simulink model "b_SCARA_4_DOF_disturbance"  (R2024b)
settings: Solver=ode45  StartTime=0.0  StopTime=8  RelTol=1e-3
libraries: sm_lib x13, nesl_utility x13
settings Model: Creator=Hamid Reza  LastModifiedBy=Hamid Reza
settings SolverCC: MaxConsecutiveZCs=50000

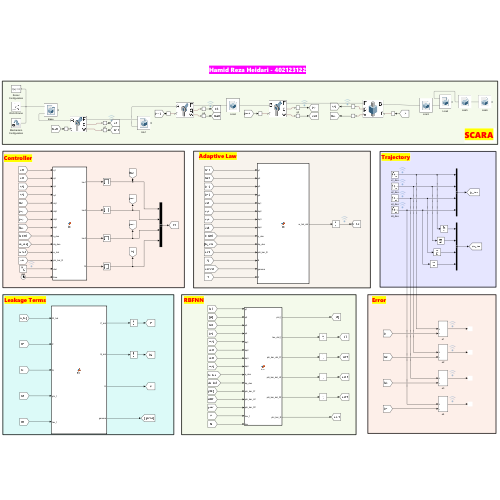
[thumbnail: Simulink's stored preview of the top-level diagram]
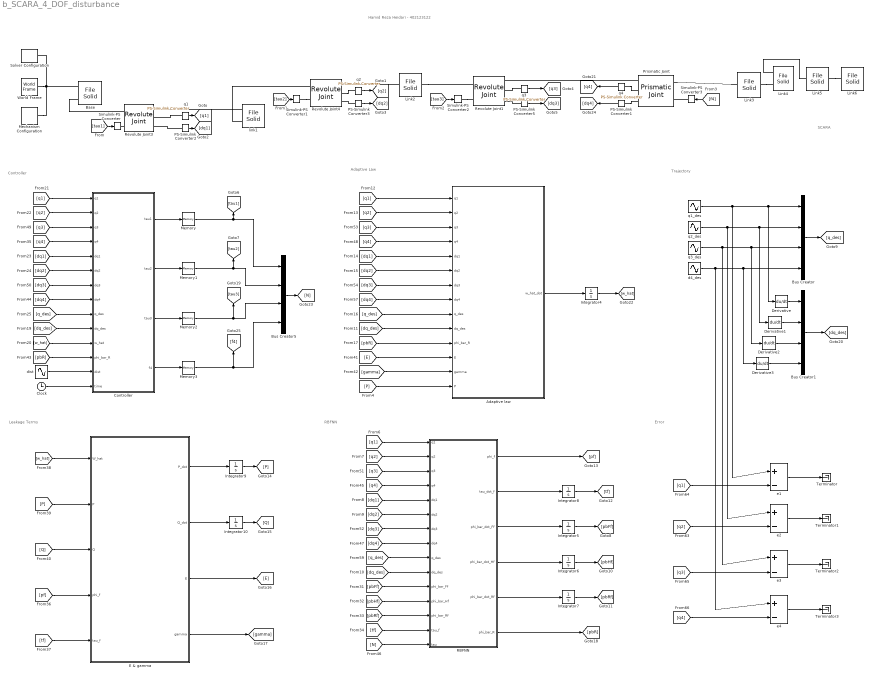
== system b_SCARA_4_DOF_disturbance ==
  note: SCARA
  note: RBFNN
  note: Controller
  note: Adaptive Law
  note: Leakage Terms
  note: Trajectory
  note: Error
  note: Hamid Reza Heidari - 402123122
  Adaptive law : MATLAB Function  TreatAsAtomicUnit=on
  Base : sm_lib/Body Elements/File Solid  ExtGeomFileName=D:\Education\ME\This Semester\Advance Robotics\HW\SimScape\Project 1\SCARA Model_SDLPRT Format\grnd.SLDPRT  UnitType=FromFile  ExtGeomFileUnits=m  StepReaderType=HEX  ExportConvexHullGeometry=off  InertiaType=CalculateFromGeometry  BasedOnType=Mass  Density=1000  DensityUnits=kg/m^3  Mass=5257.95  MassUnits=g  CenterOfMass=[0 0 0]  CenterOfMassUnits=m  MomentsOfInertia=[1 1 1]  MomentsOfInertiaUnits=kg*m^2  ProductsOfInertia=[0 0 0]  ProductsOfInertiaUnits=kg*m^2  GraphicType=FromGeometry  MarkerShape=Sphere  MarkerSize=10  GraphicVisPropType=SimpleVisualProperties  GraphicDiffuseColor=[0.5 0.5 0.5]  GraphicOpacity=1.0  GraphicSpecularColor=[0.5 0.5 0.5 1.0]  GraphicAmbientColor=[0.15 0.15 0.15 1.0]  GraphicEmissiveColor=[0.0 0.0 0.0 1.0]  GraphicShininess=75  DoExposeReferenceFrame=on  SerializedFrames=<Frames><Frame><Id>Frame1</Id><Value><Name>{0}</Name><Origin><Source>GeometricFeature</Source><FeatureName>general surface 32</FeatureName></Origin><PrimaryAxis><DefinedDirection>+X</DefinedDirection><Source>ReferenceFrame</Source><SourceDirection>-Y</SourceDirection><FeatureName></FeatureName></PrimaryAxis><SecondaryAxis><DefinedDirection>+Z</DefinedDirection><Source>ReferenceFrame</Source><SourceDirection>+Z</SourceDirection><FeatureName></FeatureName></SecondaryAxis></Value></Frame><Frame><Id>Frame2</Id><Value><Name>{1}</Name><Origin><Source>GeometricFeature</Source><FeatureName>general surface 10</FeatureName></Origin><PrimaryAxis><DefinedDirection>+Z</DefinedDirection><Source>ReferenceFrame</Source><SourceDirection>+Z</SourceDirection><FeatureName></FeatureName></PrimaryAxis><SecondaryAxis><DefinedDirection>+X</DefinedDirection><Source>ReferenceFrame</Source><SourceDirection>+X</SourceDirection><FeatureName></FeatureName></SecondaryAxis></Value></Frame></Frames>
  Bus Creator : BusCreator  Inputs=4
  Bus Creator1 : BusCreator  Inputs=4
  Bus Creator5 : BusCreator  Inputs=4
  Clock : Clock
  Controller : MATLAB Function  TreatAsAtomicUnit=on
  Derivative{,1..3} (4 alike) : Derivative
  E & gamma : MATLAB Function  TreatAsAtomicUnit=on
  Integrator10 : Integrator  InitialCondition=zeros([4 450])
  Integrator4 : Integrator  InitialCondition=zeros([4 450])  ContinuousStateAttributes='w_hat'
  Integrator5 : Integrator  InitialCondition=zeros([450 1])
  Integrator6 : Integrator  InitialCondition=zeros([450 1])
  Integrator7 : Integrator  InitialCondition=zeros([450 1])
  Integrator8 : Integrator  InitialCondition=zeros([4 1])
  Integrator9 : Integrator  InitialCondition=zeros([450 450])
  Link2 : sm_lib/Body Elements/File Solid  ExtGeomFileName=D:\Education\ME\This Semester\Advance Robotics\HW\SimScape\Project 1\SCARA Model_SDLPRT Format\link2.SLDPRT  UnitType=FromFile  ExtGeomFileUnits=m  StepReaderType=HEX  ExportConvexHullGeometry=off  InertiaType=CalculateFromGeometry  BasedOnType=Mass  Density=1000  DensityUnits=kg/m^3  Mass=5177.21  MassUnits=g  CenterOfMass=[0 0 0]  CenterOfMassUnits=m  MomentsOfInertia=[1 1 1]  MomentsOfInertiaUnits=kg*m^2  ProductsOfInertia=[0 0 0]  ProductsOfInertiaUnits=kg*m^2  GraphicType=FromGeometry  MarkerShape=Sphere  MarkerSize=10  GraphicVisPropType=SimpleVisualProperties  GraphicDiffuseColor=[0.5 0.5 0.5]  GraphicOpacity=1.0  GraphicSpecularColor=[0.5 0.5 0.5 1.0]  GraphicAmbientColor=[0.15 0.15 0.15 1.0]  GraphicEmissiveColor=[0.0 0.0 0.0 1.0]  GraphicShininess=75  DoExposeReferenceFrame=on  SerializedFrames=<Frames><Frame><Id>Frame2</Id><Value><Name>{4}</Name><Origin><Source>GeometricFeature</Source><FeatureName>circular curve 66</FeatureName></Origin><PrimaryAxis><DefinedDirection>+Z</DefinedDirection><Source>ReferenceFrame</Source><SourceDirection>+Z</SourceDirection><FeatureName></FeatureName></PrimaryAxis><SecondaryAxis><DefinedDirection>+X</DefinedDirection><Source>ReferenceFrame</Source><SourceDirection>+X</SourceDirection><FeatureName></FeatureName></SecondaryAxis></Value></Frame></Frames>
  Link3 : sm_lib/Body Elements/File Solid  ExtGeomFileName=D:\Education\ME\This Semester\Advance Robotics\HW\SimScape\Project 1\SCARA Model_SDLPRT Format\link3.SLDPRT  UnitType=FromFile  ExtGeomFileUnits=m  StepReaderType=HEX  ExportConvexHullGeometry=off  InertiaType=CalculateFromGeometry  BasedOnType=Mass  Density=1000  DensityUnits=kg/m^3  Mass=7274.75  MassUnits=g  CenterOfMass=[0 0 0]  CenterOfMassUnits=m  MomentsOfInertia=[1 1 1]  MomentsOfInertiaUnits=kg*m^2  ProductsOfInertia=[0 0 0]  ProductsOfInertiaUnits=kg*m^2  GraphicType=FromGeometry  MarkerShape=Sphere  MarkerSize=10  GraphicVisPropType=SimpleVisualProperties  GraphicDiffuseColor=[0.5 0.5 0.5]  GraphicOpacity=1.0  GraphicSpecularColor=[0.5 0.5 0.5 1.0]  GraphicAmbientColor=[0.15 0.15 0.15 1.0]  GraphicEmissiveColor=[0.0 0.0 0.0 1.0]  GraphicShininess=75  DoExposeReferenceFrame=on  SerializedFrames=<Frames><Frame><Id>Frame2</Id><Value><Name>{5}</Name><Origin><Source>GeometricFeature</Source><FeatureName>general surface 4</FeatureName></Origin><PrimaryAxis><DefinedDirection>+Z</DefinedDirection><Source>ReferenceFrame</Source><SourceDirection>-Z</SourceDirection><FeatureName></FeatureName></PrimaryAxis><SecondaryAxis><DefinedDirection>+X</DefinedDirection><Source>ReferenceFrame</Source><SourceDirection>+X</SourceDirection><FeatureName></FeatureName></SecondaryAxis></Value></Frame></Frames>
  Link4 : sm_lib/Body Elements/File Solid  ExtGeomFileName=D:\Education\ME\This Semester\Advance Robotics\HW\SimScape\Project 1\SCARA Model_SDLPRT Format\link4.SLDPRT  UnitType=FromFile  ExtGeomFileUnits=m  StepReaderType=HEX  ExportConvexHullGeometry=off  InertiaType=CalculateFromGeometry  BasedOnType=Mass  Density=1000  DensityUnits=kg/m^3  Mass=1518.25  MassUnits=g  CenterOfMass=[0 0 0]  CenterOfMassUnits=m  MomentsOfInertia=[1 1 1]  MomentsOfInertiaUnits=kg*m^2  ProductsOfInertia=[0 0 0]  ProductsOfInertiaUnits=kg*m^2  GraphicType=FromGeometry  MarkerShape=Sphere  MarkerSize=10  GraphicVisPropType=SimpleVisualProperties  GraphicDiffuseColor=[0.5 0.5 0.5]  GraphicOpacity=1.0  GraphicSpecularColor=[0.5 0.5 0.5 1.0]  GraphicAmbientColor=[0.15 0.15 0.15 1.0]  GraphicEmissiveColor=[0.0 0.0 0.0 1.0]  GraphicShininess=75  DoExposeReferenceFrame=on  SerializedFrames=<Frames><Frame><Id>Frame3</Id><Value><Name>{7}</Name><Origin><Source>GeometricFeature</Source><FeatureName>circular curve 1</FeatureName></Origin><PrimaryAxis><DefinedDirection>+Z</DefinedDirection><Source>ReferenceFrame</Source><SourceDirection>+Z</SourceDirection><FeatureName></FeatureName></PrimaryAxis><SecondaryAxis><DefinedDirection>+X</DefinedDirection><Source>ReferenceFrame</Source><SourceDirection>+X</SourceDirection><FeatureName></FeatureName></SecondaryAxis></Value></Frame><Frame><Id>Frame4</Id><Value><Name>{6}</Name><Origin><Source>GeometricFeature</Source><FeatureName>general surface 45</FeatureName></Origin><PrimaryAxis><DefinedDirection>+Z</DefinedDirection><Source>ReferenceFrame</Source><SourceDirection>+Z</SourceDirection><FeatureName></FeatureName></PrimaryAxis><SecondaryAxis><DefinedDirection>+X</DefinedDirection><Source>ReferenceFrame</Source><SourceDirection>+X</SourceDirection><FeatureName></FeatureName></SecondaryAxis></Value></Frame></Frames>
  Link5 : sm_lib/Body Elements/File Solid  ExtGeomFileName=D:\Education\ME\This Semester\Advance Robotics\HW\SimScape\Project 1\SCARA Model_SDLPRT Format\link5.SLDPRT  UnitType=FromFile  ExtGeomFileUnits=m  StepReaderType=HEX  ExportConvexHullGeometry=off  InertiaType=CalculateFromGeometry  BasedOnType=Mass  Density=1000  DensityUnits=kg/m^3  Mass=1118.05  MassUnits=g  CenterOfMass=[0 0 0]  CenterOfMassUnits=m  MomentsOfInertia=[1 1 1]  MomentsOfInertiaUnits=kg*m^2  ProductsOfInertia=[0 0 0]  ProductsOfInertiaUnits=kg*m^2  GraphicType=FromGeometry  MarkerShape=Sphere  MarkerSize=10  GraphicVisPropType=SimpleVisualProperties  GraphicDiffuseColor=[0.5 0.5 0.5]  GraphicOpacity=1.0  GraphicSpecularColor=[0.5 0.5 0.5 1.0]  GraphicAmbientColor=[0.15 0.15 0.15 1.0]  GraphicEmissiveColor=[0.0 0.0 0.0 1.0]  GraphicShininess=75  DoExposeReferenceFrame=on  SerializedFrames=<Frames><Frame><Id>Frame1</Id><Value><Name>{8}</Name><Origin><Source>GeometricFeature</Source><FeatureName>general surface 42</FeatureName></Origin><PrimaryAxis><DefinedDirection>+Z</DefinedDirection><Source>ReferenceFrame</Source><SourceDirection>+Z</SourceDirection><FeatureName></FeatureName></PrimaryAxis><SecondaryAxis><DefinedDirection>+X</DefinedDirection><Source>ReferenceFrame</Source><SourceDirection>+X</SourceDirection><FeatureName></FeatureName></SecondaryAxis></Value></Frame></Frames>
  Link6 : sm_lib/Body Elements/File Solid  ExtGeomFileName=D:\Education\ME\This Semester\Advance Robotics\HW\SimScape\Project 1\SCARA Model_SDLPRT Format\link6.SLDPRT  UnitType=FromFile  ExtGeomFileUnits=m  StepReaderType=HEX  ExportConvexHullGeometry=off  InertiaType=CalculateFromGeometry  BasedOnType=Mass  Density=1000  DensityUnits=kg/m^3  Mass=328.36  MassUnits=g  CenterOfMass=[0 0 0]  CenterOfMassUnits=m  MomentsOfInertia=[1 1 1]  MomentsOfInertiaUnits=kg*m^2  ProductsOfInertia=[0 0 0]  ProductsOfInertiaUnits=kg*m^2  GraphicType=FromGeometry  MarkerShape=Sphere  MarkerSize=10  GraphicVisPropType=SimpleVisualProperties  GraphicDiffuseColor=[0.5 0.5 0.5]  GraphicOpacity=1.0  GraphicSpecularColor=[0.5 0.5 0.5 1.0]  GraphicAmbientColor=[0.15 0.15 0.15 1.0]  GraphicEmissiveColor=[0.0 0.0 0.0 1.0]  GraphicShininess=75  DoExposeReferenceFrame=on  SerializedFrames=<Frames><Frame><Id>Frame1</Id><Value><Name>{9}</Name><Origin><Source>GeometricFeature</Source><FeatureName>general surface 9</FeatureName></Origin><PrimaryAxis><DefinedDirection>+Z</DefinedDirection><Source>ReferenceFrame</Source><SourceDirection>+Z</SourceDirection><FeatureName></FeatureName></PrimaryAxis><SecondaryAxis><DefinedDirection>+X</DefinedDirection><Source>ReferenceFrame</Source><SourceDirection>+X</SourceDirection><FeatureName></FeatureName></SecondaryAxis></Value></Frame></Frames>
  Mechanism Configuration : sm_lib/Utilities/Mechanism Configuration  UniformGravity=Constant  GravityVector=[0 0 -9.80665]  GravityVectorUnits=m/s^2  LinearizationDelta=0.001  JointModeTransitionNonlinearIterations=2
  Memory{,1..3} (4 alike) : Memory
  PS-Simulink Converter{1..3,5} (4 alike) : nesl_utility/PS-Simulink Converter  PhysicalDomain=network_engine_domain  SubClassName=ps_output  LeftPortType=input  RightPortType=output  PseudoPeriodic=off  Frequencies=[]  VectorFormat=inherit  Unit=inherit  AffineConversion=off
  Prismatic Joint : sm_lib/Joints/Prismatic Joint  JointMode=Normal  CompositeWrenchDir=FollowerOnBase  CompositeWrenchFrame=BaseFrame  SenseConstraintForce=off  SenseConstraintTorque=off  SenseTotalForce=off  SenseTotalTorque=off  PositionTargetSpecify=off  PositionTargetPriority=High  PositionTargetValue=0  PositionTargetValueUnits=m  VelocityTargetSpecify=off  VelocityTargetPriority=High  VelocityTargetValue=0  VelocityTargetValueUnits=m/s  EquilibriumPosition=0  EquilibriumPositionUnits=m  SpringStiffness=0  SpringStiffnessUnits=N/m  DampingCoefficient=0  DampingCoefficientUnits=N/(m/s)  LowerLimitSpecify=on  LowerLimitBound=0  LowerLimitBoundUnits=m  LowerLimitStiffness=1e6  LowerLimitStiffnessUnits=N/m  LowerLimitDamping=1e3  LowerLimitDampingUnits=N/(m/s)  LowerLimitTransitionRegionWidth=1e-4  LowerLimitTransitionRegionWidthUnits=m  UpperLimitSpecify=on  UpperLimitBound=0.3  UpperLimitBoundUnits=m  UpperLimitStiffness=1e6  UpperLimitStiffnessUnits=N/m  UpperLimitDamping=1e3  UpperLimitDampingUnits=N/(m/s)  UpperLimitTransitionRegionWidth=1e-4  UpperLimitTransitionRegionWidthUnits=m  TorqueActuationMode=InputTorque  MotionActuationMode=ComputedMotion  SensePosition=on  SenseVelocity=on  SenseAcceleration=off  SenseTorqueForce=off  SenseLowerLimitTorqueForce=off  SenseUpperLimitTorqueForce=off
  RBFNN : MATLAB Function  TreatAsAtomicUnit=on
  Revolute Joint1 : sm_lib/Joints/Revolute Joint  JointMode=Normal  CompositeWrenchDir=FollowerOnBase  CompositeWrenchFrame=BaseFrame  SenseConstraintForce=off  SenseConstraintTorque=off  SenseTotalForce=off  SenseTotalTorque=off  PositionTargetSpecify=off  PositionTargetPriority=High  PositionTargetValue=0  PositionTargetValueUnits=deg  VelocityTargetSpecify=off  VelocityTargetPriority=High  VelocityTargetValue=0  VelocityTargetValueUnits=deg/s  EquilibriumPosition=0  EquilibriumPositionUnits=deg  SpringStiffness=0  SpringStiffnessUnits=N*m/deg  DampingCoefficient=0  DampingCoefficientUnits=N*m/(deg/s)  LowerLimitSpecify=off  LowerLimitBound=-145  LowerLimitBoundUnits=deg  LowerLimitStiffness=1e4  LowerLimitStiffnessUnits=N*m/deg  LowerLimitDamping=10  LowerLimitDampingUnits=N*m/(deg/s)  LowerLimitTransitionRegionWidth=0.1  LowerLimitTransitionRegionWidthUnits=deg  UpperLimitSpecify=off  UpperLimitBound=145  UpperLimitBoundUnits=deg  UpperLimitStiffness=1e4  UpperLimitStiffnessUnits=N*m/deg  UpperLimitDamping=10  UpperLimitDampingUnits=N*m/(deg/s)  UpperLimitTransitionRegionWidth=0.1  UpperLimitTransitionRegionWidthUnits=deg  TorqueActuationMode=InputTorque  MotionActuationMode=ComputedMotion  SensePosition=on  SenseVelocity=on  SenseAcceleration=off  SenseTorqueForce=off  SenseLowerLimitTorqueForce=off  SenseUpperLimitTorqueForce=off
  Revolute Joint3 : sm_lib/Joints/Revolute Joint  JointMode=Normal  CompositeWrenchDir=FollowerOnBase  CompositeWrenchFrame=BaseFrame  SenseConstraintForce=off  SenseConstraintTorque=off  SenseTotalForce=off  SenseTotalTorque=off  PositionTargetSpecify=off  PositionTargetPriority=High  PositionTargetValue=0  PositionTargetValueUnits=deg  VelocityTargetSpecify=off  VelocityTargetPriority=High  VelocityTargetValue=0  VelocityTargetValueUnits=deg/s  EquilibriumPosition=0  EquilibriumPositionUnits=deg  SpringStiffness=0  SpringStiffnessUnits=N*m/deg  DampingCoefficient=0  DampingCoefficientUnits=N*m/(deg/s)  LowerLimitSpecify=on  LowerLimitBound=-125  LowerLimitBoundUnits=deg  LowerLimitStiffness=1e4  LowerLimitStiffnessUnits=N*m/deg  LowerLimitDamping=10  LowerLimitDampingUnits=N*m/(deg/s)  LowerLimitTransitionRegionWidth=0.1  LowerLimitTransitionRegionWidthUnits=deg  UpperLimitSpecify=on  UpperLimitBound=125  UpperLimitBoundUnits=deg  UpperLimitStiffness=1e4  UpperLimitStiffnessUnits=N*m/deg  UpperLimitDamping=10  UpperLimitDampingUnits=N*m/(deg/s)  UpperLimitTransitionRegionWidth=0.1  UpperLimitTransitionRegionWidthUnits=deg  TorqueActuationMode=InputTorque  MotionActuationMode=ComputedMotion  SensePosition=on  SenseVelocity=on  SenseAcceleration=off  SenseTorqueForce=off  SenseLowerLimitTorqueForce=off  SenseUpperLimitTorqueForce=off
  Revolute Joint4 : sm_lib/Joints/Revolute Joint  JointMode=Normal  CompositeWrenchDir=FollowerOnBase  CompositeWrenchFrame=BaseFrame  SenseConstraintForce=off  SenseConstraintTorque=off  SenseTotalForce=off  SenseTotalTorque=off  PositionTargetSpecify=off  PositionTargetPriority=High  PositionTargetValue=0  PositionTargetValueUnits=deg  VelocityTargetSpecify=off  VelocityTargetPriority=High  VelocityTargetValue=0  VelocityTargetValueUnits=deg/s  EquilibriumPosition=0  EquilibriumPositionUnits=deg  SpringStiffness=0  SpringStiffnessUnits=N*m/deg  DampingCoefficient=0  DampingCoefficientUnits=N*m/(deg/s)  LowerLimitSpecify=on  LowerLimitBound=-145  LowerLimitBoundUnits=deg  LowerLimitStiffness=1e4  LowerLimitStiffnessUnits=N*m/deg  LowerLimitDamping=10  LowerLimitDampingUnits=N*m/(deg/s)  LowerLimitTransitionRegionWidth=0.1  LowerLimitTransitionRegionWidthUnits=deg  UpperLimitSpecify=on  UpperLimitBound=145  UpperLimitBoundUnits=deg  UpperLimitStiffness=1e4  UpperLimitStiffnessUnits=N*m/deg  UpperLimitDamping=10  UpperLimitDampingUnits=N*m/(deg/s)  UpperLimitTransitionRegionWidth=0.1  UpperLimitTransitionRegionWidthUnits=deg  TorqueActuationMode=InputTorque  MotionActuationMode=ComputedMotion  SensePosition=on  SenseVelocity=on  SenseAcceleration=off  SenseTorqueForce=off  SenseLowerLimitTorqueForce=off  SenseUpperLimitTorqueForce=off
  Simulink-PS Converter{,1..3} (4 alike) : nesl_utility/Simulink-PS Converter  PhysicalDomain=network_engine_domain  SubClassName=ps_input  LeftPortType=input  RightPortType=output  PseudoPeriodic=off  Frequencies=[]  NoiseDistribution=none  NoiseParameters=[]  Unit=1  AffineConversion=off  FilteringAndDerivatives=provide  SimscapeFilterOrder=1  InputFilterTimeConstant=0.001  UdotUserProvided=0
  Solver Configuration : nesl_utility/Solver Configuration  PhysicalDomain=network_engine_domain  SubClassName=solver  LeftPortType=input  RightPortType=generic  Tones=[]  Harmonics=[]  SimulateNoise=off  Profile=off  UseLocalSampling=off  EnableSwitchedLinearOptims=on  FrequencyDomain=off  UseCCode=off  RelTol=0.001  AbsTol=1e-06  MinStep=1e-09  ToWorkspace=off  RevertToSquareIcSolve=off  NumHomotopyIterations=100  PhasorMode=off  PhasorModeNumHarmonics=1  ConsistencySolver=NEWTON_XTOL_AFTER_FTOL  IndexReductionMethod=DerivativeReplacement  DoDC=off  ResidualTolerance=1e-09  ConsistencyTolSource=GLOBAL  ConsistencyAbsTol=0.001  ConsistencyRelTol=0.001  ConsistencyTolFactor=0.001  UseLocalSolver=off  LocalSolverChoice=NE_BACKWARD_EULER_ADVANCER  ResolveIndetEquations=on  FunctionEvalNumThread=1  LocalSolverSampleTime=0.001  DoFixedCost=off  MaxNonlinIter=3  MaxModeIter=2  ComputeImpulses=off  ImpulseIterations=2  LinearAlgebra=Sparse  LinearAlgebraNumThread=0  EquationFormulation=NE_TIME_EF  DelaysMemoryBudget=1024  AutomaticFiltering=on  FilteringTimeConstant=0.001  PartitionStorageMethod=AS_NEEDED  PartitionMemoryBudget=1024  PartitionMethod=FAST  MultibodyUseLocalSolver=off  MultibodyLocalSolverChoice=ODE1  MultibodyLocalSolverSampleTime=0.001
  Terminator{,1..3} (4 alike) : Terminator
  World Frame : sm_lib/Frames and Transforms/World Frame
  d4_des : Sin  Amplitude=0.12  Bias=0.12  Frequency=1.5  Phase=4.88  SampleTime=0
  dist : Sin  Amplitude=8  Frequency=10  SampleTime=0
  e{1..4} (4 alike) : Sum  Inputs=|+-
  link1 : sm_lib/Body Elements/File Solid  ExtGeomFileName=D:\Education\ME\This Semester\Advance Robotics\HW\SimScape\Project 1\SCARA Model_SDLPRT Format\link1.SLDPRT  UnitType=FromFile  ExtGeomFileUnits=m  StepReaderType=HEX  ExportConvexHullGeometry=off  InertiaType=CalculateFromGeometry  BasedOnType=Mass  Density=1000  DensityUnits=kg/m^3  Mass=2195.03  MassUnits=g  CenterOfMass=[0 0 0]  CenterOfMassUnits=m  MomentsOfInertia=[1 1 1]  MomentsOfInertiaUnits=kg*m^2  ProductsOfInertia=[0 0 0]  ProductsOfInertiaUnits=kg*m^2  GraphicType=FromGeometry  MarkerShape=Sphere  MarkerSize=10  GraphicVisPropType=SimpleVisualProperties  GraphicDiffuseColor=[0.5 0.5 0.5]  GraphicOpacity=1.0  GraphicSpecularColor=[0.5 0.5 0.5 1.0]  GraphicAmbientColor=[0.15 0.15 0.15 1.0]  GraphicEmissiveColor=[0.0 0.0 0.0 1.0]  GraphicShininess=75  DoExposeReferenceFrame=on  SerializedFrames=<Frames><Frame><Id>Frame1</Id><Value><Name>{2}</Name><Origin><Source>GeometricFeature</Source><FeatureName>circular curve 48</FeatureName></Origin><PrimaryAxis><DefinedDirection>+Z</DefinedDirection><Source>ReferenceFrame</Source><SourceDirection>+Z</SourceDirection><FeatureName></FeatureName></PrimaryAxis><SecondaryAxis><DefinedDirection>+X</DefinedDirection><Source>ReferenceFrame</Source><SourceDirection>+X</SourceDirection><FeatureName></FeatureName></SecondaryAxis></Value></Frame><Frame><Id>Frame3</Id><Value><Name>{3}</Name><Origin><Source>GeometricFeature</Source><FeatureName>general surface 11</FeatureName></Origin><PrimaryAxis><DefinedDirection>+Z</DefinedDirection><Source>ReferenceFrame</Source><SourceDirection>+Z</SourceDirection><FeatureName></FeatureName></PrimaryAxis><SecondaryAxis><DefinedDirection>+X</DefinedDirection><Source>ReferenceFrame</Source><SourceDirection>+X</SourceDirection><FeatureName></FeatureName></SecondaryAxis></Value></Frame></Frames>
  q{1..4} (4 alike) : nesl_utility/PS-Simulink Converter  PhysicalDomain=network_engine_domain  SubClassName=ps_output  LeftPortType=input  RightPortType=output  PseudoPeriodic=off  Frequencies=[]  VectorFormat=inherit  Unit=inherit  AffineConversion=off
  q1_des : Sin  Amplitude=2  Frequency=3  SampleTime=0
  q2_des : Sin  Amplitude=2.24  Frequency=2.3  SampleTime=0
  q3_des : Sin  Amplitude=3.36  Frequency=2.58  SampleTime=0
  wires:
  [tau2] -> Simulink-PS Converter1/1
  q1/1 -> [q1]
  q2/1 -> [q2]
  PS-Simulink Converter2/1 -> [dq1]
  [q2] -> Controller/2(q2)
  Integrator10/1 -> [Q]
  [Q] -> E & gamma/3(Q)
  E & gamma/1(P_dot) -> Integrator9/1
  [pbFf] -> RBFNN/11(phi_bar_Ff)
  [dq1] -> RBFNN/5(dq1)
  [tf] -> RBFNN/14(tau_f)
  [q3] -> RBFNN/3(q3)
  Integrator6/1 -> [pbHf]
  [dq2] -> Adaptive law/6(dq2)
  Integrator5/1 -> [pbFf]
  [q2] -> RBFNN/2(q2)
  [dq_des] -> Controller/10(dq_des)
  [dq1] -> Controller/5(dq1)
  [gamma] -> Adaptive law/13(gamma)
  [q3] -> Adaptive law/3(q3)
  RBFNN/3(phi_bar_dot_Ff) -> Integrator5/1
  [pbR] -> Adaptive law/11(phi_bar_R)
  RBFNN/2(tau_dot_f) -> Integrator8/1
  Integrator8/1 -> [tf]
  RBFNN/1(phi_f) -> [pf]
  Integrator7/1 -> [pbRf]
  E & gamma/4(gamma) -> [gamma]
  RBFNN/4(phi_bar_dot_Hf) -> Integrator6/1
  [q_des] -> RBFNN/9(q_des)
  [w_hat] -> E & gamma/1(W_hat)
  q1_des/1 -> Derivative/1, Bus Creator/1, e1/1
  E & gamma/3(E) -> [E]
  Bus Creator1/1 -> [dq_des]
  [q1] -> RBFNN/1(q1)
  q3_des/1 -> Derivative2/1, Bus Creator/3, e3/1
  [q_des] -> Adaptive law/9(q_des)
  Adaptive law/1(w_hat_dot) -> Integrator4/1
  [E] -> Adaptive law/12(E)
  [P] -> E & gamma/2(P)
  [pbR] -> Controller/12(phi_bar_R)
  q2_des/1 -> Derivative1/1, Bus Creator/2, e2/1
  [pbHf] -> RBFNN/12(phi_bar_Hf)
  Integrator4/1 -> [w_hat]
  Bus Creator/1 -> [q_des]
  [q1] -> Adaptive law/1(q1)
  [q_des] -> Controller/9(q_des)
  [dq_des] -> Adaptive law/10(dq_des)
  RBFNN/6(phi_bar_R) -> [pbR]
  [q1] -> Controller/1(q1)
  [tf] -> E & gamma/5(tau_f)
  Integrator9/1 -> [P]
  [q3] -> Controller/3(q3)
  [q2] -> Adaptive law/2(q2)
  [dq1] -> Adaptive law/5(dq1)
  [dq3] -> Adaptive law/7(dq3)
  E & gamma/2(Q_dot) -> Integrator10/1
  [dq_des] -> RBFNN/10(dq_des)
  [w_hat] -> Controller/11(w_hat)
  [pbRf] -> RBFNN/13(phi_bar_Rf)
  [pf] -> E & gamma/4(phi_f)
  RBFNN/5(phi_bar_dot_Rf) -> Integrator7/1
  [dq2] -> RBFNN/6(dq2)
  [dq3] -> RBFNN/7(dq3)
  PS-Simulink Converter3/1 -> [dq2]
  Bus Creator5/1 -> [N]
  Controller/1(tau1) -> Memory/1
  Controller/2(tau2) -> Memory1/1
  Controller/3(tau3) -> Memory2/1
  q3/1 -> [q3]
  PS-Simulink Converter5/1 -> [dq3]
  [tau3] -> Simulink-PS Converter2/1
  [f4] -> Simulink-PS Converter3/1
  q4/1 -> [q4]
  Controller/4(f4) -> Memory3/1
  [q4] -> Controller/4(q4)
  [q4] -> Adaptive law/4(q4)
  [dq4] -> Adaptive law/8(dq4)
  d4_des/1 -> Derivative3/1, Bus Creator/4, e4/1
  [tau1] -> Simulink-PS Converter/1
  PS-Simulink Converter1/1 -> [dq4]
  [dq2] -> Controller/6(dq2)
  [dq3] -> Controller/7(dq3)
  [dq4] -> Controller/8(dq4)
  Memory1/1 -> Bus Creator5/2, [tau2]
  Memory/1 -> Bus Creator5/1, [tau1]
  Memory2/1 -> Bus Creator5/3, [tau3]
  Memory3/1 -> [f4], Bus Creator5/4
  [N] -> RBFNN/15(tau)
  [dq4] -> RBFNN/8(dq4)
  [q4] -> RBFNN/4(q4)
  Derivative/1 -> Bus Creator1/1
  Derivative1/1 -> Bus Creator1/2
  Derivative2/1 -> Bus Creator1/3
  Derivative3/1 -> Bus Creator1/4
  e1/1 -> Terminator/1
  e2/1 -> Terminator1/1
  e3/1 -> Terminator2/1
  e4/1 -> Terminator3/1
  [q1] -> e1/2
  [q2] -> e2/2
  [q4] -> e4/2
  [q3] -> e3/2
  [P] -> Adaptive law/14(P)
  Clock/1 -> Controller/14(time)
  dist/1 -> Controller/13(dist)
  connections:
  Link4/LConn1 -- Link5/LConn1
  Revolute Joint4/RConn1 -- Link2/LConn1
  Mechanism Configuration/RConn1 -- World Frame/RConn1 -- Base/LConn1 -- Solver Configuration/RConn1
  Revolute Joint3/RConn1 -- link1/LConn1
  Link3/RConn1 -- Link4/LConn2
  Base/LConn2 -- Revolute Joint3/LConn1
  Link5/RConn1 -- Link6/LConn1
  link1/LConn2 -- Revolute Joint4/LConn1
  Simulink-PS Converter1/RConn1 -- Revolute Joint4/LConn2
  q1/LConn1 -- Revolute Joint3/RConn2
  Revolute Joint4/RConn2 -- q2/LConn1
  PS-Simulink Converter2/LConn1 -- Revolute Joint3/RConn3
  PS-Simulink Converter3/LConn1 -- Revolute Joint4/RConn3
  Link2/RConn1 -- Revolute Joint1/LConn1
  q3/LConn1 -- Revolute Joint1/RConn2
  PS-Simulink Converter5/LConn1 -- Revolute Joint1/RConn3
  Simulink-PS Converter2/RConn1 -- Revolute Joint1/LConn2
  Prismatic Joint/RConn1 -- Revolute Joint1/RConn1
  Simulink-PS Converter3/RConn1 -- Prismatic Joint/LConn2
  Simulink-PS Converter/RConn1 -- Revolute Joint3/LConn2
  q4/LConn1 -- Prismatic Joint/RConn2
  PS-Simulink Converter1/LConn1 -- Prismatic Joint/RConn3
  Link3/LConn1 -- Prismatic Joint/LConn1

== matlab function b_SCARA_4_DOF_disturbance/RBFNN ==
  data: q1 input; q2 input; q3 input; q4 input; dq1 input; dq2 input; dq3 input; dq4 input; q_des input; dq_des input; phi_f output; tau_dot_f output; phi_bar_Ff input; phi_bar_Hf input; phi_bar_Rf input; phi_bar_dot_Ff output; phi_bar_dot_Hf output; phi_bar_dot_Rf output; tau_f input; phi_bar_R output; tau input
function [phi_f, tau_dot_f, phi_bar_dot_Ff, phi_bar_dot_Hf, phi_bar_dot_Rf, phi_bar_R] = fcn(q1, q2, q3, q4, dq1, dq2, dq3, dq4, q_des, dq_des, phi_bar_Ff, phi_bar_Hf, phi_bar_Rf, tau_f, tau)

N = 150;
k = 0.001;
center_range = [-4,4];
dim_z = 12;
N_center = N*3*dim_z;

de = dq_des - [dq1;dq2;dq3;dq4];
e = q_des - [q1;q2;q3;q4];

N_ZERO = zeros([N 1]);

z = [q1, q2, q3, dq1, dq2, dq3, e(1), e(2), e(3), de(1), de(2), de(3)]';

centers = linspace(center_range(1), center_range(2), N_center);

phi_F = zeros([N 1]);
phi_H = zeros([N 1]);
phi_R = zeros([N 1]);

for i = 1:1:N
    
    eta = pi;

    idx = (i-1)*(3*dim_z)+1;

    zeta_F = centers(idx:idx+dim_z-1);
    zeta_H = centers(idx+dim_z:idx+2*dim_z-1);
    zeta_R = centers(idx+2*dim_z:i+3*dim_z-1);

    phi_F(i) = phi(z, zeta_F, eta);
    phi_H(i) = phi(z, zeta_H, eta);
    phi_R(i) = phi(z, zeta_R, eta);

end

phi_bar_F = [phi_F; N_ZERO; N_ZERO];
phi_bar_H = [N_ZERO; phi_H; N_ZERO];
phi_bar_R = [N_ZERO; N_ZERO; phi_R];


phi_bar_dot_Ff = (phi_bar_F - phi_bar_Ff)/k;
phi_bar_dot_Hf = (phi_bar_H - phi_bar_Hf)/k;
phi_bar_dot_Rf = (phi_bar_R - phi_bar_Rf)/k;


phi_f = ((phi_bar_F - phi_bar_Ff)/k)+phi_bar_Hf-phi_bar_Rf;
tau_dot_f = ( tau - tau_f)/k;


end


function F = phi(z, zeta, eta)

F = exp((-1/eta)*norm(z-zeta)^2);

end

== matlab function b_SCARA_4_DOF_disturbance/Controller ==
  data: tau1 output; tau2 output; q1 input; tau3 output; q2 input; q3 input; q4 input; dq1 input; dq2 input; dq3 input; dq4 input; q_des input; dq_des input; w_hat input; phi_bar_R input; f4 output; dist input; time input
function [tau1, tau2, tau3, f4]  = fcn(q1, q2, q3, q4, dq1, dq2, dq3, dq4, q_des, dq_des, w_hat, phi_bar_R, dist, time)

K = diag([96 96 96 96]);
landa = 0.05;
K2 = diag([80 80 80 80]);
epsilon = 0.001;

de = dq_des - [dq1;dq2;dq3;dq4];
e = q_des - [q1;q2;q3;q4];
s = de + landa*e;


if norm(s) > epsilon
    X_s = K2*s/norm(s);
else
    X_s = K2*s/epsilon;
end

tau = w_hat*phi_bar_R + K*s + X_s;

if time<0.2
    tau1 = tau(1);
    tau2 = tau(2);
    tau3 = tau(3);
    f4 = tau(4);
else
    tau1 = tau(1)+dist;
    tau2 = tau(2)+dist;
    tau3 = tau(3)+dist;
    f4 = tau(4)+0.1*dist;
end

end

== matlab function b_SCARA_4_DOF_disturbance/E & gamma ==
  data: W_hat input; P_dot output; P input; Q input; Q_dot output; E output; gamma output; phi_f input; tau_f input
function [P_dot, Q_dot, E, gamma] = fcn(W_hat, P, Q, phi_f, tau_f)

l = 5;
kappa = 6;

P_dot = -l*P + kappa*phi_f*phi_f';
Q_dot = -l*Q - kappa*tau_f*phi_f';

E = W_hat*P-Q;

gamma = kappa*W_hat*phi_f*phi_f' + kappa*tau_f*phi_f';

== matlab function b_SCARA_4_DOF_disturbance/Adaptive law ==
  data: q1 input; q2 input; q3 input; q4 input; dq1 input; dq2 input; dq3 input; dq4 input; q_des input; w_hat_dot output; dq_des input; phi_bar_R input; E input; gamma input; P input
function w_hat_dot = fcn(q1, q2, q3, q4, dq1, dq2, dq3, dq4, q_des, dq_des, phi_bar_R, E, gamma, P)

GAMMA = 10;
alpha = 0.5;
beta = alpha;
landa = 0.05;
epsilon = 0.001;

de = dq_des - [dq1;dq2;dq3;dq4];
e = q_des - [q1;q2;q3;q4];
s = de + landa*e;

if norm(E) > epsilon
    smt = E*P/norm(E);
else
    smt = E*P/epsilon;
end

w_hat_dot = GAMMA*(s*phi_bar_R' - alpha*smt - beta*gamma);
